simulink model "Noh_Nofusion"  (R2020b)
settings: Solver=FixedStepAuto  StartTime=0.0  StopTime=Inf  FixedStep=0.01  RelTol=1e-3
PostLoadFcn:
  | if any(exist('dsrtsu_mdlpostloadfcn', 'file') ~= 0), dsrtsu_mdlpostloadfcn('Execute', bdroot); end
InitFcn:
  | , if any(exist('rtifpga_mdlclblib', 'file') ~= 0), rtifpga_mdlclblib('Init', bdroot); end,
  | , if any(exist('dsmpb_private', 'file') ~= 0), dsmpb_private('dsmpb_mdlclblib', 'Init', bdroot); end,
undefined symbols (not defined in the file): ACC_TimeGap_DecSetSwt, ACC_TimeGap_IncSetSwt, AccelPedalPosn, AccelPedalPosnVldty, AccelPedlPosnDiagc, AccPedalOverride, ACU_ShiftInProgress, ADAS_Posn_CurLane, AESSwtReq, ALC_SwtReq, BrkPedalSts, CC_ACC_CANCEL_OFFSwt, CC_ACC_CRUISE_OFFSwt, CC_ACC_DecSetSpd_SetSwt, CC_ACC_IncSetSpd_ResuSwt, CC_ACCSwtErr, CharSpd_ms, CSA_NODE, CURRENT_GEAR, CurrentGearValid, DiscIntNeverNeededParam, DrvDoorSts, DrvSBR, DrvTrqReqOvld, ECMACCInterface, ECMRespACC, ELKSwtReq, EngLimpHomeSts, EngSpd, EngState, EngState_PHEV, EngTrqMaxActSpd, EngTrqMinAct, EPS_DrvInpTrqVal_HighReslolution, EPS_FailSts, EPS_LKATorqOvrlDlvd, EPS_LKATorqOvrlDlvdVld, EPS_LKATrqOvlDlvdSts, EPS_SteerMod, EPS_TrqSnsrSts, EQ4_APPINFO, EQ4_LA_ELEM, EQ4_LA_HDR, EQ4_LAP_ELEM, EQ4_LAP_HDR, EQ4_LH_ELEM, EQ4_LH_HDR, EQ4_LRE_ELEM, EQ4_LRE_HDR, ESS_PedSwtReq, ESS_VehSwtReq, FFogLmpSts_F_Pbox, FLWheelDriveDirection, FLWheelSpd, FrntWiprSwtSts, FrntWshrSwtSts, FRWheelDriveDirection, FRWheelSpd, HazardLmpSwtSts, HCU_AccelPedalPosn_Diag ... (+153)
libraries: simulink x132, dsmpblib x27
(part 3 of 14)

== system Noh_Nofusion/EQ4_Lane_Pack1 ==
  In1 : Inport
  Bus Assignment : BusAssignment  AssignedSignals=LA_Zero_byte,LA_Protocol_Version,LA_Sync_ID,LA_Adjacent_Count
  Bus Assignment1 : BusAssignment  AssignedSignals=EQ4_LH_HDR,EQ4_LH_ELEM,EQ4_APPINFO.APP_SyncTs
  Bus Assignment2 : BusAssignment  AssignedSignals=EQ4_LRE_HDR,EQ4_LRE_ELEM
  Bus Assignment3 : BusAssignment  AssignedSignals=EQ4_LA_HDR,EQ4_LA_ELEM
  Bus Assignment4 : BusAssignment  AssignedSignals=LRE_Zero_byte,Reserved_1,LRE_CRC,LRE_Protocol_Version,LRE_Sync_ID,LRE_Count,LRE_Header_Buffer
  Bus Assignment5 : BusAssignment  AssignedSignals=LAP_Zero_byte,LAP_Protocol_Version,LAP_Sync_ID,LAP_Is_Construction_Area,LAP_Buffer_C0,LAP_INTP_Available,LAP_INTP_Count,LAP_Exit_Merge_Available,LAP_Is_Highway_Merge_Left,LAP_Is_Highway_Merge_Right,LAP_Is_Highway_Exit_Left,LAP_Is_Highway_Exit_Right,LAP_Vertical_Surface_Available,LAP_Vertical_Surface_VR_End,Reserved_1,LAP_Vertical_Surface_C0,LAP_Vertical_Surface_C1,LAP_Vertical_Surface_C2,LAP_Vertical_Surface_C3,LAP_Path_Pred_CRC,LAP_Path_Pred_Available,LAP_Path_Pred_First_Valid,LAP_Path_Pred_Second_Valid,LAP_Path_Pred_Half_Width,LAP_Path_Pred_Conf,LAP_Is_Triggered_SDM_Model,Reserved_2,LAP_Path_Pred_First_VR_End,LAP_Path_Pred_second_VR_End,Reserved_3,LAP_Path_Pred_First_C0,LAP_Path_Pred_First_C1,LAP_Path_Pred_First_C2,LAP_Path_Pred_First_C3,LAP_Path_Pred_Second_C0,LAP_Path_Pred_Second_C1,LAP_Path_Pred_Second_C2,LAP_Path_Pred_Second_C3
  Bus Assignment6 : BusAssignment  AssignedSignals=LH_Zero_byte,LH_Protocol_Version,LH_Sync_ID,LH_Lanes_Count,Reserved_1,LH_Estimated_Width,Reserved_2
  Bus Assignment7 : BusAssignment  AssignedSignals=EQ4_LAP_HDR,EQ4_LAP_ELEM
  Bus Selector : BusSelector  OutputSignals=EQ4_LA.EQ4_LA_HDR,EQ4_LA.EQ4_LA_ELEM,EQ4_LA.EQ4_APPINFO.H
  Bus Selector1 : BusSelector  OutputSignals=EQ4_LH.EQ4_LH_HDR,EQ4_LH.EQ4_LH_ELEM,EQ4_LH.EQ4_APPINFO.H
  Bus Selector2 : BusSelector  OutputSignals=EQ4_LRE.EQ4_LRE_HDR,EQ4_LRE.EQ4_LRE_ELEM,EQ4_LRE.EQ4_APPINFO.H
  Bus Selector3 : BusSelector  OutputSignals=LA_Zero_byte,LA_Protocol_Version,LA_Sync_ID,LA_Adjacent_Count
  Bus Selector4 : BusSelector  OutputSignals=LRE_Zero_byte,Reserved_1,LRE_CRC,LRE_Protocol_Version,LRE_Sync_ID,LRE_Count,LRE_Header_Buffer
  Bus Selector5 : BusSelector  OutputSignals=LH_Zero_byte,LH_Protocol_Version,LH_Sync_ID,LH_Lanes_Count,Reserved_1,LH_Estimated_Width,Reserved_2
  Bus Selector6 : BusSelector  OutputSignals=EQ4_LAP.EQ4_LAP_HDR,EQ4_LAP.EQ4_LAP_ELEM,EQ4_LAP.EQ4_APPINFO.H
  Bus Selector7 : BusSelector  OutputSignals=LAP_Zero_byte,LAP_Protocol_Version,LAP_Sync_ID,LAP_Is_Construction_Area,LAP_Buffer_C0,LAP_INTP_Available,LAP_INTP_Count,LAP_Exit_Merge_Available,LAP_Is_Highway_Merge_Left,LAP_Is_Highway_Merge_Right,LAP_Is_Highway_Exit_Left,LAP_Is_Highway_Exit_Right,LAP_Vertical_Surface_Available,LAP_Vertical_Surface_VR_End,Reserved_1,LAP_Vertical_Surface_C0,LAP_Vertical_Surface_C1,LAP_Vertical_Surface_C2,LAP_Vertical_Surface_C3,LAP_Path_Pred_CRC,LAP_Path_Pred_Available,LAP_Path_Pred_First_Valid,LAP_Path_Pred_Second_Valid,LAP_Path_Pred_Half_Width,LAP_Path_Pred_Conf,LAP_Is_Triggered_SDM_Model,Reserved_2,LAP_Path_Pred_First_VR_End,LAP_Path_Pred_second_VR_End,Reserved_3,LAP_Path_Pred_First_C0,LAP_Path_Pred_First_C1,LAP_Path_Pred_First_C2,LAP_Path_Pred_First_C3,LAP_Path_Pred_Second_C0,LAP_Path_Pred_Second_C1,LAP_Path_Pred_Second_C2,LAP_Path_Pred_Second_C3
  Constant1 : Constant  Value=0  OutDataTypeStr=Bus: EQ4_LA_BUS
  Constant2 : Constant  Value=0  OutDataTypeStr=Bus: EQ4_LH_BUS
  Constant3 : Constant  Value=0  OutDataTypeStr=Bus: EQ4_LRE_BUS
  Constant4 : Constant  Value=0  OutDataTypeStr=Bus: EQ4_LA_HDR_BUS
  Constant5 : Constant  Value=0  OutDataTypeStr=Bus: EQ4_LRE_HDR_BUS
  Constant6 : Constant  Value=0  OutDataTypeStr=Bus: EQ4_LAP_BUS
  Constant7 : Constant  Value=0  OutDataTypeStr=Bus: EQ4_LH_HDR_BUS
  Constant8 : Constant  Value=0  OutDataTypeStr=Bus: EQ4_LAP_HDR_BUS
  Data Type Conversion{,1..4} (5 alike) : DataTypeConversion
  For Each Subsystem1 : Subsystem  TreatAsAtomicUnit=on
  For Each Subsystem2 : Subsystem  TreatAsAtomicUnit=on
  For Each Subsystem3 : Subsystem  TreatAsAtomicUnit=on
  For Each Subsystem4 : Subsystem  TreatAsAtomicUnit=on
  EQ4_LAP : Outport
  EQ4_LA : Outport  Port=2
  EQ4_LH : Outport  Port=3
  EQ4_LRE : Outport  Port=4
  wires:
  In1/1 -> Bus Selector2/1, Bus Selector1/1, Bus Selector6/1, Bus Selector/1
  Bus Assignment2/1 -> EQ4_LRE/1  "mcuEQ4_LRE"
  Constant2/1 -> Bus Assignment1/1
  Bus Assignment1/1 -> EQ4_LH/1  "mcuEQ4_LH"
  Constant3/1 -> Bus Assignment2/1
  Bus Assignment3/1 -> EQ4_LA/1  "mcuEQ4_LA"
  Bus Selector/1 -> Bus Selector3/1  "<EQ4_LA_HDR>"
  Bus Selector/2 -> For Each Subsystem3/1(In1)  "<EQ4_LA_ELEM>"
  Bus Selector1/1 -> Bus Selector5/1  "<EQ4_LH_HDR>"
  Bus Selector1/2 -> For Each Subsystem1/1(In1)  "<EQ4_LH_ELEM>"
  Bus Selector2/1 -> Bus Selector4/1  "<EQ4_LRE_HDR>"
  Bus Selector2/2 -> For Each Subsystem2/1(In1)  "<EQ4_LRE_ELEM>"
  Constant1/1 -> Bus Assignment3/1
  Constant4/1 -> Bus Assignment/1
  Bus Assignment/1 -> Bus Assignment3/2
  Bus Selector3/1 -> Bus Assignment/2  "<LA_Zero_byte>"
  Bus Selector3/2 -> Bus Assignment/3  "<LA_Protocol_Version>"
  Bus Selector3/4 -> Bus Assignment/5  "<LA_Adjacent_Count>"
  Constant5/1 -> Bus Assignment4/1
  Bus Selector4/6 -> Bus Assignment4/7  "<LRE_Count>"
  Bus Selector4/7 -> Bus Assignment4/8  "<LRE_Header_Buffer>"
  Bus Selector4/4 -> Bus Assignment4/5  "<LRE_Protocol_Version>"
  Bus Selector4/3 -> Bus Assignment4/4  "<LRE_CRC>"
  Bus Selector4/2 -> Bus Assignment4/3  "<Reserved_1>"
  Bus Selector4/1 -> Bus Assignment4/2  "<LRE_Zero_byte>"
  Bus Assignment4/1 -> Bus Assignment2/2
  Constant7/1 -> Bus Assignment6/1
  Bus Assignment6/1 -> Bus Assignment1/2
  Bus Selector5/6 -> Bus Assignment6/7  "<LH_Estimated_Width>"
  Bus Selector5/5 -> Bus Assignment6/6  "<Reserved_1>"
  Bus Selector5/7 -> Bus Assignment6/8  "<Reserved_2>"
  Bus Selector5/4 -> Bus Assignment6/5  "<LH_Lanes_Count>"
  Bus Selector5/2 -> Bus Assignment6/3  "<LH_Protocol_Version>"
  Bus Selector5/1 -> Bus Assignment6/2  "<LH_Zero_byte>"
  For Each Subsystem1/1(Out1) -> Bus Assignment1/3
  For Each Subsystem2/1(Out1) -> Bus Assignment2/3
  For Each Subsystem3/1(Out1) -> Bus Assignment3/3
  Bus Selector1/3 -> Data Type Conversion2/1, Data Type Conversion/1  "<H>"
  Data Type Conversion/1 -> Bus Assignment1/4
  Bus Selector/3 -> Data Type Conversion1/1  "<H>"
  Data Type Conversion1/1 -> Bus Assignment/4
  Data Type Conversion2/1 -> Bus Assignment6/4
  Data Type Conversion3/1 -> Bus Assignment4/6
  Bus Selector2/3 -> Data Type Conversion3/1  "<H>"
  Data Type Conversion4/1 -> Bus Assignment5/4
  For Each Subsystem4/1(Out1) -> Bus Assignment7/3
  Bus Assignment5/1 -> Bus Assignment7/2
  Constant8/1 -> Bus Assignment5/1
  Constant6/1 -> Bus Assignment7/1
  Bus Selector6/2 -> For Each Subsystem4/1(In1)  "<EQ4_LAP_ELEM>"
  Bus Assignment7/1 -> EQ4_LAP/1  "mcuEQ4_LAP"
  Bus Selector6/3 -> Data Type Conversion4/1  "<H>"
  Bus Selector6/1 -> Bus Selector7/1  "<EQ4_LAP_HDR>"
  Bus Selector7/1 -> Bus Assignment5/2  "<LAP_Zero_byte>"
  Bus Selector7/2 -> Bus Assignment5/3  "<LAP_Protocol_Version>"
  Bus Selector7/4 -> Bus Assignment5/5  "<LAP_Is_Construction_Area>"
  Bus Selector7/5 -> Bus Assignment5/6  "<LAP_Buffer_C0>"
  Bus Selector7/6 -> Bus Assignment5/7  "<LAP_INTP_Available>"
  Bus Selector7/7 -> Bus Assignment5/8  "<LAP_INTP_Count>"
  Bus Selector7/8 -> Bus Assignment5/9  "<LAP_Exit_Merge_Available>"
  Bus Selector7/9 -> Bus Assignment5/10  "<LAP_Is_Highway_Merge_Left>"
  Bus Selector7/10 -> Bus Assignment5/11  "<LAP_Is_Highway_Merge_Right>"
  Bus Selector7/11 -> Bus Assignment5/12  "<LAP_Is_Highway_Exit_Left>"
  Bus Selector7/12 -> Bus Assignment5/13  "<LAP_Is_Highway_Exit_Right>"
  Bus Selector7/13 -> Bus Assignment5/14  "<LAP_Vertical_Surface_Available>"
  Bus Selector7/14 -> Bus Assignment5/15  "<LAP_Vertical_Surface_VR_End>"
  Bus Selector7/15 -> Bus Assignment5/16  "<Reserved_1>"
  Bus Selector7/16 -> Bus Assignment5/17  "<LAP_Vertical_Surface_C0>"
  Bus Selector7/17 -> Bus Assignment5/18  "<LAP_Vertical_Surface_C1>"
  Bus Selector7/18 -> Bus Assignment5/19  "<LAP_Vertical_Surface_C2>"
  Bus Selector7/19 -> Bus Assignment5/20  "<LAP_Vertical_Surface_C3>"
  Bus Selector7/20 -> Bus Assignment5/21  "<LAP_Path_Pred_CRC>"
  Bus Selector7/21 -> Bus Assignment5/22  "<LAP_Path_Pred_Available>"
  Bus Selector7/22 -> Bus Assignment5/23  "<LAP_Path_Pred_First_Valid>"
  Bus Selector7/23 -> Bus Assignment5/24  "<LAP_Path_Pred_Second_Valid>"
  Bus Selector7/24 -> Bus Assignment5/25  "<LAP_Path_Pred_Half_Width>"
  Bus Selector7/25 -> Bus Assignment5/26  "<LAP_Path_Pred_Conf>"
  Bus Selector7/26 -> Bus Assignment5/27  "<LAP_Is_Triggered_SDM_Model>"
  Bus Selector7/27 -> Bus Assignment5/28  "<Reserved_2>"
  Bus Selector7/28 -> Bus Assignment5/29  "<LAP_Path_Pred_First_VR_End>"
  Bus Selector7/29 -> Bus Assignment5/30  "<LAP_Path_Pred_second_VR_End>"
  Bus Selector7/30 -> Bus Assignment5/31  "<Reserved_3>"
  Bus Selector7/31 -> Bus Assignment5/32  "<LAP_Path_Pred_First_C0>"
  Bus Selector7/32 -> Bus Assignment5/33  "<LAP_Path_Pred_First_C1>"
  Bus Selector7/33 -> Bus Assignment5/34  "<LAP_Path_Pred_First_C2>"
  Bus Selector7/34 -> Bus Assignment5/35  "<LAP_Path_Pred_First_C3>"
  Bus Selector7/35 -> Bus Assignment5/36  "<LAP_Path_Pred_Second_C0>"
  Bus Selector7/36 -> Bus Assignment5/37  "<LAP_Path_Pred_Second_C1>"
  Bus Selector7/37 -> Bus Assignment5/38  "<LAP_Path_Pred_Second_C2>"
  Bus Selector7/38 -> Bus Assignment5/39  "<LAP_Path_Pred_Second_C3>"

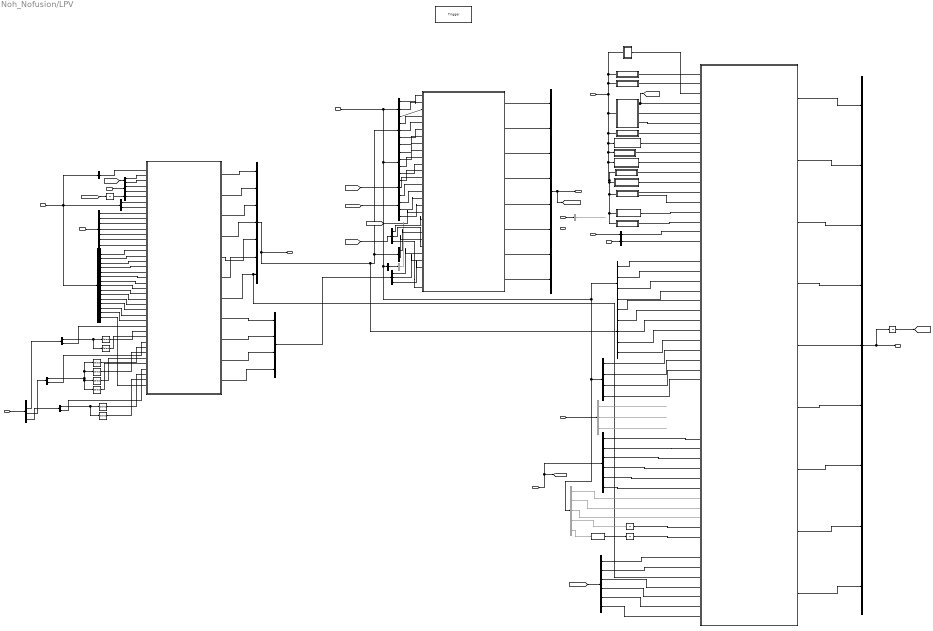
== system Noh_Nofusion/LPV ==
  FaultRnk : Inport
  FaultTriggers : Inport  Port=2
  IfALLBus : Inport  Port=3
  IfCANBus : Inport  Port=4
  IfCALBus : Inport  Port=5
  IfDMSBus : Inport  Port=6
  IfEHRBus : Inport  Port=7
  IfVIEBus : Inport  Port=8
  IfEQ4Bus : Inport  Port=9
  RFM_LANES : Inport  Port=10
  function : TriggerPort  TriggerType=function-call  VariantControl=Variant
  ABM_Pack : Subsystem
  BCM_Pack : Subsystem
  Bus Creator : BusCreator  Inputs=9
  Bus Creator1 : BusCreator  Inputs=8
  Bus Creator3 : BusCreator  Inputs=4
  Bus Creator9 : BusCreator  Inputs=7
  Bus Selector : BusSelector  OutputSignals=LSM_UpdateCnt,LSM_TJA_ICA,LSM_HWA,LSM_LCK,LSM_ESS
  Bus Selector1 : BusSelector  OutputSignals=signal1.TOS_P0_TARGET_LINE
  Bus Selector10 : BusSelector  OutputSignals=LSM_HWA,LSM_ESS,LSM_UpdateCnt
  Bus Selector12 : BusSelector  OutputSignals=VSM_LON_CTRL
  Bus Selector13 : BusSelector  OutputSignals=LSM_PilotSPLDist,LSM_PilotSPL,LSM_PilotRoadSts
  Bus Selector14 : BusSelector  OutputSignals=PLAN_ALC_DECS
  Bus Selector15 : BusSelector  OutputSignals=EQ4_LA_ELEM,EQ4_LA_HDR
  Bus Selector16 : BusSelector  OutputSignals=PLAN_ACCPLAN,PLAN_DriverOffConditionFulfilled,PLAN_ALC_DECS,PLAN_DPC_ESS,PLAN_NOH_SetSpdAdjReq,PLAN_NOH_SetSpdAdjVal
  Bus Selector17 : BusSelector  OutputSignals=EQ4_LH_ELEM,EQ4_LH_HDR
  Bus Selector18 : BusSelector  OutputSignals=VSM_HMI,VSM_UOM_LC_BUS,MRCReq
  Bus Selector19 : BusSelector  OutputSignals=DriverSts
  Bus Selector2 : BusSelector  OutputSignals=vxvRefMs,kapTraj
  Bus Selector20 : BusSelector  OutputSignals=CAL_VSM_CONFIG
  Bus Selector21 : BusSelector  OutputSignals=lanebus.RFM_LINE_L1,lanebus.RFM_LINE_R1,lanebus.RFM_LINE_LB,lanebus.RFM_LINE_RB
  Bus Selector22 : BusSelector  Commented=on  OutputSignals=EHRV2_HDR,EHRV2_ROAD_ROI,EHRV2_ROAD_INFO
  Bus Selector23 : BusSelector  OutputSignals=axvRefMs2,vxvRefMs,axvRoadSlopeMs2,axRefDt,ayvRefMs2,kapTraj
  Bus Selector24 : BusSelector  Commented=on  OutputSignals=aebbus.AEB_IPHUT_INFO,aebbus.AEB_BRK_INFO,roadbus.RFM_TSR,latbus.LATC_IFCAngCmdReqValue,latbus.LATC_IFCFuncAngCmdReqFlag
  Bus Selector25 : BusSelector  OutputSignals=signal1.TOS_ACCP0,signal1.TOS_AEB_LONOBJ,signal1.TOS_ELK,signal1.TOS_LCKIE
  Bus Selector26 : BusSelector  OutputSignals=EQ4_LRE_ELEM,EQ4_LRE_HDR
  Bus Selector27 : BusSelector  OutputSignals=lanebus.RFM_LINE_L1,lanebus.RFM_LINE_R1,roadbus.RFM_TSR
  Bus Selector28 : BusSelector  Commented=on  OutputSignals=LONC_VLC_InternalAcc
  Bus Selector29 : BusSelector  OutputSignals=LSM_PilotSts,LSM_PilotTurnSwSts
  Bus Selector3 : BusSelector  OutputSignals=lanebus.RFM_LINE_L1,lanebus.RFM_LINE_R1,lanebus.RFM_LINE_L2,lanebus.RFM_LINE_R2,lanebus.RFM_LINE_L3,lanebus.RFM_LINE_R3,lanebus.RFM_LINE_CL,lanebus.RFM_LINE_LB,lanebus.RFM_LINE_RB,lanebus.RFM_LINE_PRED,lanebus.RFM_LINEF_LB,lanebus.RFM_LINEF_RB,lanebus.RFM_LINE_ENTRY_CL,lanebus.RFM_LINE_EXIT_CL,roadbus.RFM_TSR
  Bus Selector30 : BusSelector  OutputSignals=lonbus
  Bus Selector31 : BusSelector  OutputSignals=RFM_BRANCH_LANE,RFM_LEFT_LANE,RFM_CURRENT_LANE,RFM_RIGHT_LANE,RFM_INTERSEC_ALERT,RFM_BRANCH,RFM_REC_LANES
  Bus Selector4 : BusSelector  OutputSignals=VSM_HMI,MRCReq
  Bus Selector5 : BusSelector  OutputSignals=roadbus.RFM_ROAD,roadbus.RFM_UpdateCnt
  Bus Selector6 : BusSelector  OutputSignals=signal1.TOS_LC,signal1.TOS_ACCP0,signal1.TOS_ACCP1,signal1.TOS_ACCP2,signal1.TOS_ACCP3,signal1.TOS_UpdateCnt
  Bus Selector7 : BusSelector  OutputSignals=vxvRefMs,axvRefMs2,axvRoadSlopeMs2,kapTraj
  Bus Selector8 : BusSelector  OutputSignals=EQ4_LAP,EQ4_LH,EQ4_LA,EQ4_LRE
  Bus Selector9 : BusSelector  Commented=on  OutputSignals=DFIM_VSM_STS
  CSA_Pack : Subsystem
  DCT_Pack : Subsystem
  Data Type Conversion : DataTypeConversion  OutDataTypeStr=uint8
  ECM_Pack : Subsystem
  ESP_Pack : Subsystem
  HAP_Pack : Subsystem
  HUT_Pack : Subsystem
  IfALLBus1 : InportShadow  Port=3
  IfVIEBus1 : InportShadow  Port=8
  PLAN : ModelReference  ModelNameDialog=PubIfDecisionPLAN_MDL.slx  SimulationMode=Normal  ModelReferenceVersion=1.156
  Selector : Selector  InputPortWidth=4  IndexOptions=Index vector (dialog)  Indices=1  OutputSizes=1
  Selector1 : Selector  InputPortWidth=4  IndexOptions=Index vector (dialog)  Indices=2  OutputSizes=1
  Selector2 : Selector  InputPortWidth=4  IndexOptions=Index vector (dialog)  Indices=3  OutputSizes=1
  Selector3 : Selector  InputPortWidth=4  IndexOptions=Index vector (dialog)  Indices=4  OutputSizes=1
  Selector4 : Selector  InputPortWidth=2  IndexOptions=Index vector (dialog)  Indices=1  OutputSizes=1
  Selector5 : Selector  InputPortWidth=2  IndexOptions=Index vector (dialog)  Indices=2  OutputSizes=1
  Selector6 : Selector  InputPortWidth=2  IndexOptions=Index vector (dialog)  Indices=1  OutputSizes=1
  Selector7 : Selector  InputPortWidth=2  IndexOptions=Index vector (dialog)  Indices=2  OutputSizes=1
  Subsystem : Subsystem
  Subsystem1 : Subsystem
  Subsystem2 : Subsystem
  Subsystem3 : Subsystem
  Subsystem4 : Subsystem
  Subsystem5 : Subsystem
  Unit Delay{1..4} (4 alike) : UnitDelay  SampleTime=-1  HasFrameUpgradeWarning=on
  VSM : Subsystem
  IfVSMBus : Outport
  IfLSMBus : Outport  Port=2
  IfPlanbus : Outport  Port=3
  wires:
  Bus Selector4/2 -> Subsystem5/3(VSM_ReqMRC)  "<MRCReq>"
  Bus Selector18/3 -> PLAN/29  "<MRCReq>"
  Data Type Conversion/1 -> Unit Delay2/1
  Bus Selector3/15 -> Subsystem5/41(RFM_TSR)  "<RFM_TSR>"
  Selector7/1 -> Subsystem5/40(EQ4_LRE_ELEM1)
  Selector6/1 -> Subsystem5/39(EQ4_LRE_ELEM)
  Bus Selector26/1 -> Selector6/1, Selector7/1  "<EQ4_LRE_ELEM>"
  Bus Selector26/2 -> Subsystem5/38(EQ4_LRE_HDR)  "<EQ4_LRE_HDR>"
  Selector3/1 -> Subsystem5/37(EQ4_LA_ELEM3)
  Selector2/1 -> Subsystem5/36(EQ4_LA_ELEM2)
  Selector1/1 -> Subsystem5/35(EQ4_LA_ELEM1)
  Selector/1 -> Subsystem5/34(EQ4_LA_ELEM)
  Selector5/1 -> Subsystem5/32(EQ4_LH_ELEM1)
  Selector4/1 -> Subsystem5/31(EQ4_LH_ELEM)
  Bus Selector17/2 -> Subsystem5/30(EQ4_LH_HDR)  "<EQ4_LH_HDR>"
  Bus Selector17/1 -> Selector4/1, Selector5/1  "<EQ4_LH_ELEM>"
  Bus Selector8/2 -> Bus Selector17/1  "<EQ4_LH>"
  Bus Selector15/2 -> Subsystem5/33(EQ4_LA_HDR)  "<EQ4_LA_HDR>"
  Bus Selector15/1 -> Selector2/1, Selector3/1, Selector1/1, Selector/1  "<EQ4_LA_ELEM>"
  Subsystem4/1(Out1) -> VSM/3(VSM_VCAN_HCU)
  Subsystem2/1(<HighBeamSts_HC>) -> VSM/15(VSM_VCAN_HC)
  HUT_Pack/2(VSM_VCAN_CR) -> VSM/14(VSM_VCAN_CR)
  Subsystem1/1(<IP_VehSpdUnit>) -> VSM/12(VSM_VCAN_IP)
  Subsystem/1(<ACAmbTemp>) -> VSM/8(VSM_ACAmbTemp)
  ESP_Pack/3(VSM_VCAN_PEPS) -> VSM/6(VSM_VCAN_PEPS)
  ESP_Pack/2(VSM_VCAN_EPS) -> VSM/5(VSM_VCAN_EPS)
  Bus Selector13/3 -> PLAN/26  "<LSM_PilotRoadSts>"
  Bus Selector16/6 -> VSM/56(PLAN_NOH_SetSpdAdjVal)  "<PLAN_NOH_SetSpdAdjVal>"
  Bus Selector16/5 -> VSM/55(PLAN_NOH_SetSpdAdjReq)  "<PLAN_NOH_SetSpdAdjReq>"
  PLAN/8 -> Bus Creator1/8  "PLAN_NOH_SetSpdAdjVal"
  PLAN/7 -> Bus Creator1/7  "PLAN_NOH_SetSpdAdjReq"
  Bus Selector13/2 -> PLAN/25  "<LSM_PilotSPL>"
  Bus Selector13/1 -> PLAN/24  "<LSM_PilotSPLDist>"
  Bus Creator3/1 -> Bus Selector13/1
  Subsystem5/11(LSM_PilotRoadSts) -> Bus Creator3/4  "LSM_PilotRoadSts"
  Subsystem5/10(LSM_PilotSPL) -> Bus Creator3/3
  Subsystem5/9(LSM_PilotSPLDist) -> Bus Creator3/2
  Subsystem5/8(LSM_PilotNohExitDist) -> Bus Creator3/1
  Bus Selector16/1 -> VSM/50(PLAN_ACCPLAN)  "<PLAN_ACCPLAN>"
  Bus Selector16/2 -> VSM/51(PLAN_DriverOffConditionFulfilled)  "<PLAN_DriverOffConditionFulfilled>"
  Bus Selector16/3 -> VSM/53(PLAN_ALC_Decision)  "<PLAN_ALC_DECS>"
  Bus Selector16/4 -> VSM/54(PLAN_DPC_ESS)  "<PLAN_DPC_ESS>"
  PLAN/6 -> Bus Creator1/6
  PLAN/5 -> Bus Creator1/5
  PLAN/4 -> Bus Creator1/4  "PLAN_HMI"
  [ESP_Pack] -> PLAN/18
  Bus Selector28/1 -> PLAN/20  "<LONC_VLC_InternalAcc>"
  Bus Selector29/2 -> PLAN/22  "<LSM_PilotTurnSwSts>"
  Bus Selector29/1 -> PLAN/21  "<LSM_PilotSts>"
  Bus Selector3/14 -> Subsystem5/29(RFM_LINE_EXIT_CL)  "<RFM_LINE_EXIT_CL>"
  Bus Selector3/13 -> Subsystem5/28(RFM_LINE_ENTRY_CL)  "<RFM_LINE_ENTRY_CL>"
  Bus Selector3/12 -> Subsystem5/27(RFM_LINEF_RB)  "<RFM_LINEF_RB>"
  Bus Selector3/11 -> Subsystem5/26(RFM_LINEF_LB)  "<RFM_LINEF_LB>"
  Bus Selector3/10 -> Subsystem5/25(RFM_LINE_PRED)  "<RFM_LINE_PRED>"
  Bus Selector3/9 -> Subsystem5/24(RFM_LINE_RB)  "<RFM_LINE_RB>"
  Bus Selector3/8 -> Subsystem5/23(RFM_LINE_LB)  "<RFM_LINE_LB>"
  Bus Selector3/7 -> Subsystem5/22(RFM_LINE_CL)  "<RFM_LINE_CL>"
  Bus Selector3/6 -> Subsystem5/21(RFM_LINE_R3)  "<RFM_LINE_R3>"
  Bus Selector3/5 -> Subsystem5/20(RFM_LINE_L3)  "<RFM_LINE_L3>"
  Bus Selector3/4 -> Subsystem5/19(RFM_LINE_R2)  "<RFM_LINE_R2>"
  Bus Selector3/3 -> Subsystem5/18(RFM_LINE_L2)  "<RFM_LINE_L2>"
  Bus Selector3/2 -> Subsystem5/17(RFM_LINE_R1)  "<RFM_LINE_R1>"
  Bus Selector3/1 -> Subsystem5/16(RFM_LINE_L1)  "<RFM_LINE_L1>"
  Bus Selector31/7 -> Subsystem5/15(RFM_REC_LANES)  "<RFM_REC_LANES>"
  Bus Selector31/6 -> Subsystem5/14(RFM_BRANCH)  "<RFM_BRANCH>"
  Bus Selector31/5 -> Subsystem5/13(RFM_INTERSEC_ALERT)  "<RFM_INTERSEC_ALERT>"
  Bus Selector31/4 -> Subsystem5/12(RFM_RIGHT_LANE)  "<RFM_RIGHT_LANE>"
  Bus Selector31/1 -> Subsystem5/9(RFM_BRANCH_LANE)  "<RFM_BRANCH_LANE>"
  Bus Selector31/3 -> Subsystem5/11(RFM_CURRENT_LANE)  "<RFM_CURRENT_LANE>"
  Bus Selector31/2 -> Subsystem5/10(RFM_LEFT_LANE)  "<RFM_LEFT_LANE>"
  Bus Selector5/1 -> Subsystem5/7(RFM_ROAD)  "<RFM_ROAD>"
  Bus Selector5/2 -> Subsystem5/8(RFM_UpdateCnt)  "<RFM_UpdateCnt>"
  Bus Selector2/2 -> Subsystem5/5(kapTraj)  "<kapTraj>"
  Bus Selector2/1 -> Subsystem5/4(vxvRefMs)  "<vxvRefMs>"
  Bus Selector8/4 -> Bus Selector26/1  "<EQ4_LRE>"
  Bus Selector8/3 -> Bus Selector15/1  "<EQ4_LA>"
  RFM_LANES/1 -> Bus Selector31/1
  Bus Selector18/2 -> PLAN/23  "<VSM_UOM_LC_BUS>"
  Bus Selector18/1 -> PLAN/19  "<VSM_HMI>"
  Subsystem5/7(LSM_PilotSts) -> Bus Creator9/7, VSM/52(LSM_PilotSts)  "LSM_PilotSts"
  IfALLBus/1 -> Bus Selector27/1, Bus Selector6/1, Bus Selector21/1, Bus Selector25/1, Bus Selector24/1, Bus Selector30/1
  Subsystem5/6(LSM_PilotTurnSwSts) -> Bus Creator9/6  "LSM_PilotTurnSwSts"
  Bus Selector7/4 -> PLAN/17  "<kapTraj>"
  Bus Selector7/3 -> PLAN/16  "<axvRoadSlopeMs2>"
  Bus Selector7/2 -> PLAN/15  "<axvRefMs2>"
  Bus Selector7/1 -> PLAN/14  "<vxvRefMs>"
  Bus Selector30/1 -> Bus Selector28/1  "<lonbus>"
  Bus Selector12/1 -> PLAN/13  "<VSM_LON_CTRL>"
  Bus Selector27/3 -> PLAN/3  "<RFM_TSR>"
  Bus Selector6/6 -> PLAN/12  "<TOS_UpdateCnt>"
  Bus Selector6/5 -> PLAN/11  "<TOS_ACCP3>"
  Bus Selector6/4 -> PLAN/10  "<TOS_ACCP2>"
  Bus Selector6/3 -> PLAN/9  "<TOS_ACCP1>"
  Bus Selector6/2 -> PLAN/8  "<TOS_ACCP0>"
  Bus Selector6/1 -> PLAN/7  "<TOS_LC>"
  Bus Selector10/3 -> PLAN/6  "<LSM_UpdateCnt>"
  Bus Selector10/2 -> PLAN/5  "<LSM_ESS>"
  Bus Selector10/1 -> PLAN/4  "<LSM_HWA>"
  Bus Selector27/2 -> PLAN/2  "<RFM_LINE_R1>"
  Bus Selector27/1 -> PLAN/1  "<RFM_LINE_L1>"
  [IfVSMBus] -> Bus Selector18/1
  [IfPlanbus] -> Bus Selector16/1
  Unit Delay4/1 -> [IfVSMBus]
  Bus Selector14/1 -> Subsystem5/6(PLAN_ALC_DECS)  "<PLAN_ALC_DECS>"
  Unit Delay3/1 -> Bus Selector14/1
  [IfPlanbus] -> Unit Delay3/1
  Bus Creator1/1 -> [IfPlanbus], IfPlanbus/1
  PLAN/3 -> Bus Creator1/3
  PLAN/2 -> Bus Creator1/2  "PLAN_ALC_DECS"
  PLAN/1 -> Bus Creator1/1  "PLAN_DPC_ESS"
  IfEHRBus/1 -> Bus Selector22/1
  [IfVSMBus] -> Bus Selector12/1
  [IfVIEBus] -> Bus Selector7/1
  Subsystem3/1(VSM_VCAN_PBOX) -> VSM/9(VSM_VCAN_PBOX)
  BCM_Pack/1(VSM_VCAN_BCM) -> VSM/7(VSM_VCAN_BCM)
  DCT_Pack/1(VSM_VCAN_DCT) -> VSM/2(VSM_VCAN_DCT)
  ECM_Pack/1(VSM_VCAN_ECM) -> VSM/1(VSM_VCAN_ECM)
  CSA_Pack/1(VSM_VCAN_CSA) -> VSM/10(VSM_VCAN_CSA)
  ABM_Pack/1(VSM_VCAN_ABM) -> VSM/11(VSM_VCAN_ABM)
  HUT_Pack/1(VSM_VCAN_HUT) -> VSM/13(VSM_VCAN_HUT)
  HAP_Pack/1(VSM_VCAN_HAP) -> VSM/16(VSM_VCAN_HAP)
  Unit Delay2/1 -> VSM/48(LATC_IFCFuncTrqCmdReqFlag)
  Unit Delay1/1 -> VSM/47(LATC_IFCTrqOvlCmdReqValue)
  Bus Selector24/3 -> VSM/46(RFM_TSR)  "<RFM_TSR>"
  Bus Selector24/2 -> VSM/45(AEB_BRK_INFO)  "<AEB_BRK_INFO>"
  Bus Selector24/1 -> VSM/44(AEB_IPHUT_INFO)  "<AEB_IPHUT_INFO>"
  Bus Selector23/6 -> VSM/43(kapTraj)  "<kapTraj>"
  Bus Selector23/5 -> VSM/42(ayvRefMs2)  "<ayvRefMs2>"
  Bus Selector23/4 -> VSM/41(psiDtOpt)  "<axRefDt>"
  Bus Selector23/3 -> VSM/40(axvRoadSlopeMs2)  "<axvRoadSlopeMs2>"
  Bus Selector23/2 -> VSM/39(vxvRefMs)  "<vxvRefMs>"
  Bus Selector23/1 -> VSM/38(axvRefMs2)  "<axvRefMs2>"
  Bus Selector22/3 -> ?  "<EHRV2_ROAD_INFO>"
  Bus Selector22/2 -> ?  "<EHRV2_ROAD_ROI>"
  Bus Selector22/1 -> ?  "<EHRV2_HDR>"
  Bus Selector25/4 -> VSM/32(TOS_LCKIE)  "<TOS_LCKIE>"
  Bus Selector25/3 -> VSM/31(TOS_ELK)  "<TOS_ELK>"
  Bus Selector25/2 -> VSM/30(TOS_AEB_LONOBJ)  "<TOS_AEB_LONOBJ>"
  Bus Selector25/1 -> VSM/29(TOS_ACCP0)  "<TOS_ACCP0>"
  Bus Selector/5 -> VSM/28(LSM_ESS)  "<LSM_ESS>"
  Bus Selector/4 -> VSM/27(LSM_LCK)  "<LSM_LCK>"
  Bus Selector/3 -> VSM/26(LSM_HWA)  "<LSM_HWA>"
  Bus Selector/2 -> VSM/25(LSM_TJA_ICA)  "<LSM_TJA_ICA>"
  Bus Selector/1 -> VSM/24(LSM_UpdateCnt)  "<LSM_UpdateCnt>"
  Bus Selector21/4 -> VSM/23(RFM_LINE_RB)  "<RFM_LINE_RB>"
  Bus Selector21/3 -> VSM/22(RFM_LINE_LB)  "<RFM_LINE_LB>"
  Bus Selector21/2 -> VSM/21(RFM_LINE_R1)  "<RFM_LINE_R1>"
  Bus Selector21/1 -> VSM/20(RFM_LINE_L1)  "<RFM_LINE_L1>"
  Bus Selector19/1 -> VSM/17(DriverSts)  "<DriverSts>"
  ESP_Pack/1(VSM_VCAN_ESP) -> [ESP_Pack], VSM/4(VSM_VCAN_ESP)
  IfVIEBus1/1 -> Bus Selector2/1
  [IfVSMBus] -> Bus Selector4/1
  Subsystem5/5(LSM_UpdateCnt) -> Bus Creator9/5  "LSM_UpdateCnt"
  Subsystem5/4(LSM_ESS) -> Bus Creator9/4  "LSM_ESS"
  Bus Creator9/1 -> IfLSMBus/1, Bus Selector/1, Bus Selector29/1, Bus Selector10/1  "IfLSMBus"
  IfALLBus1/1 -> Bus Selector1/1, Bus Selector5/1, Bus Selector3/1
  Subsystem5/3(LSM_HWA) -> Bus Creator9/3  "LSM_HWA"
  IfEQ4Bus/1 -> Bus Selector8/1
  Bus Selector4/1 -> Subsystem5/2(VSM_HMI)  "<VSM_HMI>"
  Subsystem5/2(LSM_LCK) -> Bus Creator9/2  "LSM_LCK"
  Bus Selector1/1 -> Subsystem5/1(TOS_P0_TARGET_LINE)  "<TOS_P0_TARGET_LINE>"
  Subsystem5/1(LSM_TJA_ICA) -> Bus Creator9/1  "LSM_TJA_ICA"
  Bus Selector24/5 -> Data Type Conversion/1  "<LATC_IFCFuncAngCmdReqFlag>"
  Bus Selector24/4 -> Unit Delay1/1  "<LATC_IFCAngCmdReqValue>"
  IfVIEBus/1 -> Bus Selector23/1, [IfVIEBus]
  Bus Selector9/1 -> ?  "<DFIM_VSM_STS>"
  Bus Selector20/1 -> VSM/18(CAL_VSM_CONFIG)  "<CAL_VSM_CONFIG>"
  IfCALBus/1 -> Bus Selector20/1
  IfDMSBus/1 -> Bus Selector19/1
  IfCANBus/1 -> ESP_Pack/1(In1), BCM_Pack/1(In1), Subsystem/1(In1), ABM_Pack/1(In1), Subsystem2/1(In1), HAP_Pack/1(In1), HUT_Pack/1(In1), Subsystem1/1(In1), CSA_Pack/1(In1), Subsystem3/1(In1), ECM_Pack/1(In1), Subsystem4/1(In1), DCT_Pack/1(In1)
  FaultTriggers/1 -> Bus Selector9/1
  Bus Creator/1 -> Unit Delay4/1, IfVSMBus/1
  VSM/1(VSM_LON_CTRL) -> Bus Creator/1  "VSM_LON_CTRL"
  VSM/2(VSM_LAT_CTRL) -> Bus Creator/2  "VSM_LAT_CTRL"
  VSM/3(VSM_HMI) -> Bus Creator/3  "VSM_HMI"
  VSM/4(VSM_CTRL_LINE) -> Bus Creator/4  "VSM_CTRL_LINE"
  VSM/5(VSM_TSR) -> Bus Creator/5  "VSM_TSR"
  VSM/6(VSM_TSR_REMAIN) -> Bus Creator/6  "VSM_TSR_REMAIN"
  VSM/7(VSM_UOM_LC) -> Bus Creator/7  "VSM_UOM_LC_BUS"
  VSM/8(DataCLCT) -> Bus Creator/8  "DangerPlausMatrixVSM_HMI"
  VSM/9(VSM_MRCReq) -> Bus Creator/9  "MRCReq"

== system Noh_Nofusion/SimBCM ==
  VCAN : Inport
  PLAN_ALC_DECS : Inport  Port=2
  function : TriggerPort  TriggerType=function-call  VariantControl=Variant
  BCMsim : MATLAB Function  TreatAsAtomicUnit=on
  Bus Selector : BusSelector  OutputSignals=PLAN_ALC_DECS.PLAN_ALC_TurnLightReq
  Bus Selector3 : BusSelector  OutputSignals=CSA_NODE.CSA2_MSG.SteerWheelAngSign,CSA_NODE.CSA2_MSG.SteerWheelAng,CSA_NODE.CSA1_MSG.LTurnLmpSwtSts,CSA_NODE.CSA1_MSG.RTurnLmpSwtSts
  CSALampCtrlSim : Subsystem
  LTurnLmpSwtSts : Outport
  RTurnLmpSwtSts : Outport  Port=2
  CSASim_IDC_L2_LampReq : Outport  Port=3
  wires:
  VCAN/1 -> Bus Selector3/1
  Bus Selector3/1 -> CSALampCtrlSim/1(SteerWheelAng)  "<SteerWheelAngSign>"
  Bus Selector3/4 -> CSALampCtrlSim/4(RiLmp)  "<RTurnLmpSwtSts>"
  Bus Selector3/2 -> CSALampCtrlSim/2(SteerWheelAngSign)  "<SteerWheelAng>"
  Bus Selector3/3 -> CSALampCtrlSim/3(LeLmp)  "<LTurnLmpSwtSts>"
  PLAN_ALC_DECS/1 -> Bus Selector/1
  BCMsim/1(CSASim_LampReq) -> CSASim_IDC_L2_LampReq/1
  Bus Selector/1 -> BCMsim/3(Model_IDC_L2_LampReq), CSALampCtrlSim/5(IDC_L2_LampReq)  "<PLAN_ALC_TurnLightReq>"
  CSALampCtrlSim/2(RTurnLmpSwtSts) -> BCMsim/2(SimRiLmp), RTurnLmpSwtSts/1
  CSALampCtrlSim/1(LTurnLmpSwtSts) -> BCMsim/1(SimLeLmp), LTurnLmpSwtSts/1

== system Noh_Nofusion/Subsystem1 ==
  l3_RFMResult : Inport
  RFM_Road : Inport  Port=2
  lane : Inport  Port=3
  Bus Assignment5 : BusAssignment  AssignedSignals=RFM_ROAD.nLaneNum,RFM_ROAD.b_toll,RFM_ROAD.i_mapvalid,RFM_TSR.RoadType
  Bus Assignment6 : BusAssignment  AssignedSignals=RFM_INTERSEC_ALERT.b_is_available,RFM_INTERSEC_ALERT.f_distance,RFM_INTERSEC_ALERT.en_direction,RFM_INTERSEC_ALERT.en_type,RFM_BRANCH.f_turning_angle,RFM_BRANCH.en_RoadClass,RFM_CURRENT_LANE.en_lane_type,RFM_RIGHT_LANE.en_lane_type
  Bus Selector : BusSelector  OutputSignals=b_is_available,f_distance,en_direction,en_type,st_branch.f_turning_angle
  Bus Selector1 : BusSelector  OutputSignals=i_lane_number
  Bus Selector2 : BusSelector  OutputSignals=st_intersec_alert,st_road_info,st_lanes
  Bus Selector3 : BusSelector  OutputSignals=en_road_type,ast_lane_number_vec,b_toll
  Bus Selector5 : BusSelector  OutputSignals=en_lane_type
  Bus Selector8 : BusSelector  OutputSignals=en_lane_type
  Constant : Constant  Value=P_RFM_mapvalid
  Constant4 : Constant  Value=P_RFM_RoadType  OutDataTypeStr=uint8
  Selector1 : Selector  InputPortWidth=3  IndexOptions=Index vector (dialog)  Indices=1  OutputSizes=1
  Selector5 : Selector  InputPortWidth=3  IndexOptions=Index vector (dialog)  Indices=2  OutputSizes=1
  Selector6 : Selector  InputPortWidth=3  IndexOptions=Index vector (dialog)  Indices=3  OutputSizes=1
  IfRFM_LANES_In : Outport
  roadbus : Outport  Port=2
  wires:
  Bus Selector2/1 -> Bus Selector/1  "<st_intersec_alert>"
  Bus Selector/5 -> Bus Assignment6/6  "<f_turning_angle>"
  Bus Selector3/3 -> Bus Assignment5/3  "<b_toll>"
  Selector5/1 -> Bus Selector5/1
  Bus Selector1/1 -> Bus Assignment5/2  "<i_lane_number>"
  Bus Selector/1 -> Bus Assignment6/2  "<b_is_available>"
  Bus Selector2/3 -> Selector6/1, Selector5/1  "<st_lanes>"
  Bus Selector3/1 -> Bus Assignment6/7  "<en_road_type>"
  Bus Selector2/2 -> Bus Selector3/1  "<st_road_info>"
  Selector6/1 -> Bus Selector8/1
  Bus Assignment5/1 -> roadbus/1  "RFM_ROAD"
  Bus Selector/4 -> Bus Assignment6/5  "<en_type>"
  Bus Assignment6/1 -> IfRFM_LANES_In/1
  Bus Selector/2 -> Bus Assignment6/3  "<f_distance>"
  Bus Selector/3 -> Bus Assignment6/4  "<en_direction>"
  l3_RFMResult/1 -> Bus Selector2/1
  lane/1 -> Bus Assignment6/1
  Bus Selector5/1 -> Bus Assignment6/8  "<en_lane_type>"
  Bus Selector8/1 -> Bus Assignment6/9  "<en_lane_type>"
  Bus Selector3/2 -> Selector1/1  "<ast_lane_number_vec>"
  Selector1/1 -> Bus Selector1/1
  Constant/1 -> Bus Assignment5/4
  RFM_Road/1 -> Bus Assignment5/1
  Constant4/1 -> Bus Assignment5/5

== system Noh_Nofusion/Subsystem2 ==
  IfStateMBus : Inport
  IfVIEBus : Inport  Port=2
  IfVCAN : Inport  Port=3  OutDataTypeStr=Bus: VCAN_BUS
  visMsg : Inport  Port=4
  function : TriggerPort  TriggerType=function-call  VariantControl=Variant
  ACCOSM : Subsystem
  Bus Selector16 : BusSelector  Commented=on  OutputSignals=VSM_HMI.LCKSts,VSM_LAT_CTRL
  Bus Selector17 : BusSelector  Commented=on  OutputSignals=VSM_LON_CTRL.ACC_TimeGapSet,VSM_LON_CTRL.ACCSts
  Counter Free-Running : simulink/Sources/Counter Free-Running  NumBits=3  tsamp=-1
  Data Type Conversion : DataTypeConversion
  TOS_ACCP0 : Outport  OutDataTypeStr=Bus: TOS_ACCP0_BUS
  TOS_ACCP1 : Outport  Port=2  OutDataTypeStr=Bus: TOS_ACCP1_BUS  PortDimensions=1  BusOutputAsStruct=on
  ACCP2 : Outport  Port=3  OutDataTypeStr=Bus: TOS_ACCP2_BUS
  ACCP3 : Outport  Port=4  OutDataTypeStr=Bus: TOS_ACCP3_BUS
  TOS_ACCP4 : Outport  Port=5  OutDataTypeStr=Bus: TOS_ACCP4_BUS  PortDimensions=1  BusOutputAsStruct=on
  TOS_ACCP5 : Outport  Port=6  OutDataTypeStr=Bus: TOS_ACCP5_BUS  PortDimensions=1  BusOutputAsStruct=on
  TOS_ELK : Outport  Port=7  OutDataTypeStr=Bus: TOS_ELK_BUS  PortDimensions=1  BusOutputAsStruct=on
  TOS_LCKIE : Outport  Port=8  OutDataTypeStr=Bus: TOS_LCKIE_BUS  PortDimensions=1  BusOutputAsStruct=on
  TOS_AEB_LONOBJ : Outport  Port=9  OutDataTypeStr=Bus: TOS_AEB_LONOBJ_BUS  PortDimensions=1  BusOutputAsStruct=on
  TOS_AEB_LATOBJ : Outport  Port=10  OutDataTypeStr=Bus: TOS_AEB_LATOBJ_BUS  PortDimensions=10  BusOutputAsStruct=on
  TOS_AEB_JAOBJ : Outport  Port=11  OutDataTypeStr=Bus: TOS_AEB_JAOBJ_BUS  PortDimensions=32  BusOutputAsStruct=on
  TOS_P0_TARGET_LINE : Outport  Port=12  OutDataTypeStr=Bus: TOS_P0_TARGET_LINE_BUS
  TOS_UpdateCnt : Outport  Port=13  OutDataTypeStr=uint32  PortDimensions=1  BusOutputAsStruct=on
  wires:
  Data Type Conversion/1 -> TOS_UpdateCnt/1
  Counter Free-Running/1 -> Data Type Conversion/1
  ACCOSM/4(ACCP3) -> ACCP3/1
  ACCOSM/3(ACCP2) -> ACCP2/1
  ACCOSM/2(TEM_P0_TARGET_LINE) -> TOS_P0_TARGET_LINE/1  "TOS_P0_TARGET_LINE"
  ACCOSM/1(ACCP0) -> TOS_ACCP0/1  "TOS_ACCP0"
  IfVCAN/1 -> ACCOSM/5(VCAN)
  Bus Selector17/1 -> ACCOSM/2(TimeGap)  "<ACC_TimeGapSet>"
  Bus Selector17/2 -> ACCOSM/3(ACCMode)  "<ACCSts>"
  Bus Selector16/2 -> ACCOSM/7(desLane)  "<VSM_LAT_CTRL>"
  IfStateMBus/1 -> Bus Selector17/1, Bus Selector16/1
  visMsg/1 -> ACCOSM/1(visMsg)
  Bus Selector16/1 -> ACCOSM/6(LCKSts)  "<LCKSts>"
  IfVIEBus/1 -> ACCOSM/4(VIE)

== system Noh_Nofusion/Subsystem3 ==
  function : TriggerPort  TriggerType=function-call  VariantControl=Variant
  Compare To Constant : simulink/Logic and Bit Operations/Compare To Constant  relop===  const=1344  OutDataTypeStr=boolean
  S-Function1 : S-Function  FunctionName=sfun_roadfus_L3  SFunctionDeploymentMode=off  EnableBusSupport=off
  Subsystem2 : Subsystem
  UDP Receive (3) : dsmpblib/Data Inport  Priority=10000
      settings: SourceProductName=dSPACE Model Interface Blockset
  Out2 : Outport
  wires:
  Compare To Constant/1 -> Subsystem2/Enable
  Subsystem2/1(Out1) -> S-Function1/1
  UDP Receive (3)/3 -> Compare To Constant/1
  UDP Receive (3)/1 -> Subsystem2/1(In1)
  S-Function1/1 -> Out2/1
